simulink model "wariant1"  (R2021b)
settings: Solver=VariableStepAuto  StartTime=0.0  StopTime=10.0  RelTol=1e-3
values from neighbouring files (symbols this model uses):
  start_x = [0 0 0]    [stp01.m]
  Tp = 0.5    [stp01.m]
undefined symbols (not defined in the file or in its folder): A_1, C_1
settings Model: Creator=USER  LastModifiedBy=USER

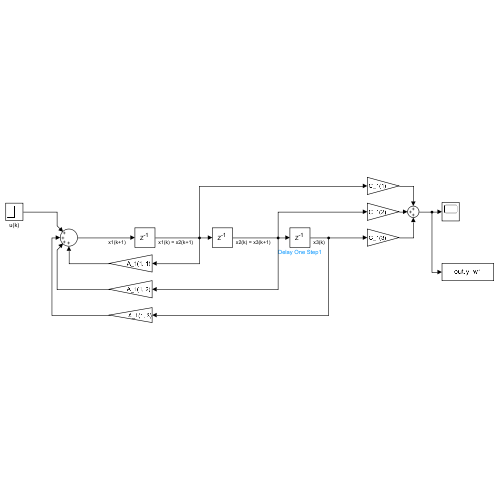
[thumbnail: Simulink's stored preview of the top-level diagram]
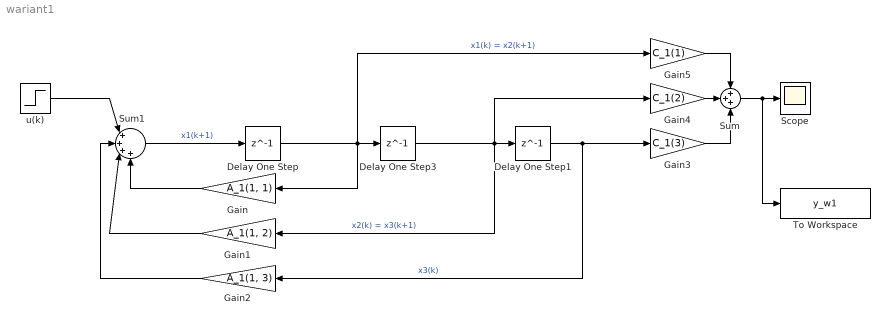
== system wariant1 ==
  Delay One Step : Delay  DelayLength=1  InitialCondition=start_x(1)  SampleTime=Tp
  Delay One Step1 : Delay  DelayLength=1  InitialCondition=start_x(3)  SampleTime=Tp
  Delay One Step3 : Delay  DelayLength=1  InitialCondition=start_x(2)  SampleTime=Tp
  Gain : Gain  Gain=A_1(1, 1)
  Gain1 : Gain  Gain=A_1(1, 2)
  Gain2 : Gain  Gain=A_1(1, 3)
  Gain3 : Gain  Gain=C_1(3)
  Gain4 : Gain  Gain=C_1(2)
  Gain5 : Gain  Gain=C_1(1)
  Scope : Scope
  Sum : Sum  Inputs=+++
  Sum1 : Sum  Inputs=|++++
  To Workspace : ToWorkspace  VariableName=y_w1  SaveFormat=Structure With Time  SampleTime=Tp
  u(k) : Step  SampleTime=Tp
  wires:
  Sum1/1 -> Delay One Step/1  "x1(k+1)"
  Delay One Step/1 -> Gain5/1, Gain/1, Delay One Step3/1  "x1(k) = x2(k+1)"
  Delay One Step3/1 -> Gain4/1, Gain1/1, Delay One Step1/1  "x2(k) = x3(k+1)"
  Delay One Step1/1 -> Gain3/1, Gain2/1  "x3(k)"
  Gain/1 -> Sum1/4
  Gain1/1 -> Sum1/3
  Gain2/1 -> Sum1/2
  u(k)/1 -> Sum1/1
  Gain3/1 -> Sum/3
  Gain4/1 -> Sum/2
  Gain5/1 -> Sum/1
  Sum/1 -> To Workspace/1, Scope/1
